simulink model "mathematical_model"  (R2022b)
settings: Solver=VariableStepAuto  StartTime=0.0  StopTime=10.0  RelTol=1e-3
libraries: simulink_extras x1
settings Model: Creator=User  LastModifiedBy=User

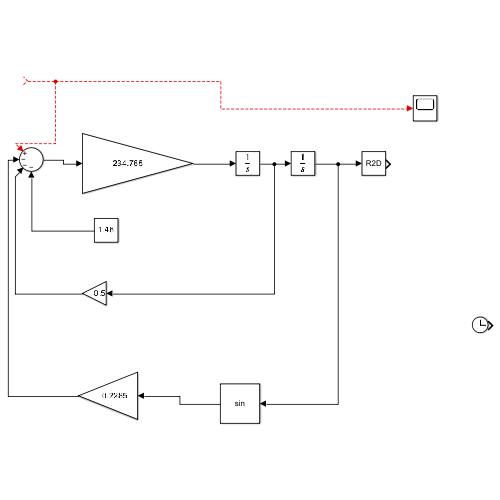
[thumbnail: Simulink's stored preview of the top-level diagram]
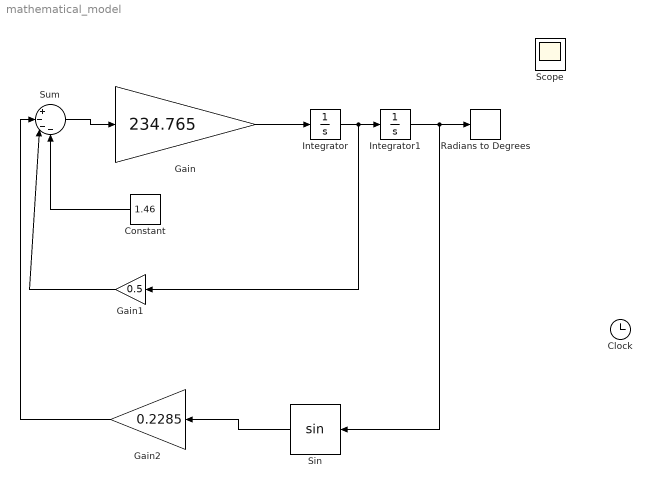
== system mathematical_model ==
  Clock : Clock
  Constant : Constant  Value=1.46
  Gain : Gain  Gain=234.765
  Gain1 : Gain  Gain=0.5
  Gain2 : Gain  Gain=0.2285
  Integrator : Integrator
  Integrator1 : Integrator
  Radians to Degrees : simulink_extras/Transformations/Radians to Degrees
  Scope : Scope
  Sin : Trigonometry
  Sum : Sum  Inputs=|+---
  wires:
  Constant/1 -> Sum/4
  Integrator/1 -> Gain1/1, Integrator1/1
  Gain/1 -> Integrator/1
  Gain1/1 -> Sum/3
  Sum/1 -> Gain/1
  Integrator1/1 -> Sin/1, Radians to Degrees/1
  Sin/1 -> Gain2/1
  Gain2/1 -> Sum/2
  ? -> Scope/1, Sum/1
